simulink model "power_machines_KLFN"  (R2014a)
settings: Solver=ode23tb  SolverMode=SingleTasking  StartTime=0.0  StopTime=60  RelTol=1e-4
libraries: powerlib x17, simulink x3, spsAC1AModel x3, powerlib_meascontrol x1
Description:
  | Copyright 2008-2014 The MathWorks, Inc.
settings Model: FPTRunName=Active  ExtModeTrigMode=oneshot  ExtModeArmWhenConnect=off  ExtModeAutoUpdateStatusClock=off  Creator=MathWorks  LastModifiedBy=jdlara
settings SolverCC: ZeroCrossAlgorithm=Adaptive
settings DataIOCC: LimitDataPoints=off  SignalLoggingSaveFormat=ModelDataLogs  SignalLoggingName=sigsOut  OutputTimes=[0:1/20:10]
settings OptimizationCC: BlockReduction=off  BooleanDataType=off  ExpressionDepthLimit=2147483647  InitFltsAndDblsToZero=on  EfficientMapNaN2IntZero=off
settings DebuggingCC: UnderspecifiedInitializationDetection=Classic  CheckExecutionContextPreStartOutputMsg=on  CheckExecutionContextRuntimeOutputMsg=on  SignalResolutionControl=TryResolveAllWithWarning  IgnoredZcDiagnostic=none  SolverPrmCheckMsg=none  MultiTaskDSMMsg=warning  MultiTaskCondExecSysMsg=none  SigSpecEnsureSampleTimeMsg=none  FcnCallInpInsideContextMsg=UseLocalSettings  UnconnectedInputMsg=none  UnconnectedOutputMsg=none  UnconnectedLineMsg=none  StateNameClashWarn=warning
settings HardwareCC: ProdHWDeviceType=Specified  TargetUnknown=on
settings RTWCC: IncludeERTFirstTime=on
settings CodeAppCC: IgnoreCustomStorageClasses=off
settings GRTTargetCC: TargetFcnLib=ansi_tfl_tmw.mat  CombineOutputUpdateFcns=off  GRTInterface=on

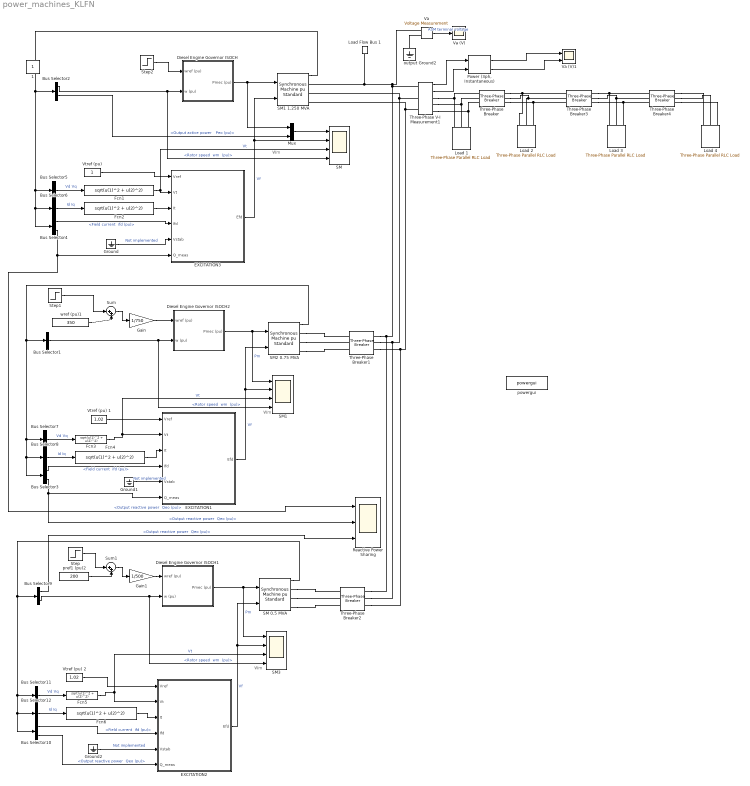
== system power_machines_KLFN ==
  note: Wm
  note: Wm
  note: Wm
  Bus Selector1 : BusSelector  OutputSignals="Mechanical.Rotor speed  wm  (pu)"
  Bus Selector10 : BusSelector  OutputSignals="dq0 components.Field current  ifd (pu),Output reactive power  Qeo (pu)"
  Bus Selector11 : BusSelector  OutputSignals="dq0 components.Stator voltage  vd (pu),dq0 components.Stator voltage  vq (pu)"  OutputAsBus=on
  Bus Selector12 : BusSelector  OutputSignals="dq0 components.Stator current  id (pu),dq0 components.Stator current  iq (pu)"  OutputAsBus=on
  Bus Selector2 : BusSelector  OutputSignals="Mechanical.Rotor speed  wm  (pu),Output active power   Peo (pu)"
  Bus Selector3 : BusSelector  OutputSignals="dq0 components.Field current  ifd (pu),Output reactive power  Qeo (pu)"
  Bus Selector4 : BusSelector  OutputSignals="dq0 components.Field current  ifd (pu),Output reactive power  Qeo (pu)"
  Bus Selector5 : BusSelector  OutputSignals="dq0 components.Stator voltage  vd (pu),dq0 components.Stator voltage  vq (pu)"  OutputAsBus=on
  Bus Selector6 : BusSelector  OutputSignals="dq0 components.Stator current  id (pu),dq0 components.Stator current  iq (pu)"  OutputAsBus=on
  Bus Selector7 : BusSelector  OutputSignals="dq0 components.Stator voltage  vd (pu),dq0 components.Stator voltage  vq (pu)"  OutputAsBus=on
  Bus Selector8 : BusSelector  OutputSignals="dq0 components.Stator current  id (pu),dq0 components.Stator current  iq (pu)"  OutputAsBus=on
  Bus Selector9 : BusSelector  OutputSignals="Output reactive power  Qeo (pu),Mechanical.Rotor speed  wm  (pu)"
  Diesel Engine Governor ISOCH : Subsystem  mask(Diesel Engine & Governor){K=5, Tr=[0.018 0.001 0.38], Ta=[0.35 0.002 0.015], Tlim=[0 1.2], Td=0.024, Pm0=0.58197}
      mask prompts: K "Regulator gain K:"; Tr "Regulator time constants [T1 T2 T3 ] (s) :"; Ta "Actuator time constants [T4 T5 T6] (s) :"; Tlim "Torque limits [Tmin Tmax] (pu) :"; Td "Engine time delay Td (s) :"; Pm0 "Initial value of mechanical power  Pm0 (pu) :"
      mask help:
      | This block implements a diesel engine and governor system:
      | 1st and 2nd inputs: Desired and actual speed (pu)
      | Output: Diesel engine mechanical power.Motor inertia should be combined with generator.
      | Controller transfer function:
      |      Hc=K.(1+T3.s)/(1+T1.s+T1.T2.s^2)
      | Actuator transfer function :
      |      Ha= (1+T4.s) / [ (s (1+T5.s)(1+T6.s) ]
      | Motor :
      |      Time delay Td
      |
      | (See reference in Tutorial Session 5)
  Diesel Engine Governor ISOCH1 : Subsystem  mask(Diesel Engine & Governor){K=5, Tr=[0.018 0.001 0.38], Ta=[0.35 0.002 0.015], Tlim=[0 1.2], Td=0.024, Pm0=0.40148}
      mask prompts: K "Regulator gain K:"; Tr "Regulator time constants [T1 T2 T3 ] (s) :"; Ta "Actuator time constants [T4 T5 T6] (s) :"; Tlim "Torque limits [Tmin Tmax] (pu) :"; Td "Engine time delay Td (s) :"; Pm0 "Initial value of mechanical power  Pm0 (pu) :"
      mask help:
      | This block implements a diesel engine and governor system:
      | 1st and 2nd inputs: Desired and actual speed (pu)
      | Output: Diesel engine mechanical power.Motor inertia should be combined with generator.
      | Controller transfer function:
      |      Hc=K.(1+T3.s)/(1+T1.s+T1.T2.s^2)
      | Actuator transfer function :
      |      Ha= (1+T4.s) / [ (s (1+T5.s)(1+T6.s) ]
      | Motor :
      |      Time delay Td
      |
      | (See reference in Tutorial Session 5)
  Diesel Engine Governor ISOCH2 : Subsystem  mask(Diesel Engine & Governor){K=5, Tr=[0.018 0.001 0.38], Ta=[0.35 0.002 0.015], Tlim=[0 1.2], Td=0.024, Pm0=0.46784}
      mask prompts: K "Regulator gain K:"; Tr "Regulator time constants [T1 T2 T3 ] (s) :"; Ta "Actuator time constants [T4 T5 T6] (s) :"; Tlim "Torque limits [Tmin Tmax] (pu) :"; Td "Engine time delay Td (s) :"; Pm0 "Initial value of mechanical power  Pm0 (pu) :"
      mask help:
      | This block implements a diesel engine and governor system:
      | 1st and 2nd inputs: Desired and actual speed (pu)
      | Output: Diesel engine mechanical power.Motor inertia should be combined with generator.
      | Controller transfer function:
      |      Hc=K.(1+T3.s)/(1+T1.s+T1.T2.s^2)
      | Actuator transfer function :
      |      Ha= (1+T4.s) / [ (s (1+T5.s)(1+T6.s) ]
      | Motor :
      |      Time delay Td
      |
      | (See reference in Tutorial Session 5)
  EXCITATION1 : Subsystem  Variant=on  OverrideUsingVariant=Variant1
      settings: AttributesFormatString=%<BlockChoice>
  EXCITATION2 : Subsystem  Variant=on  OverrideUsingVariant=Variant1
      settings: AttributesFormatString=%<BlockChoice>
  EXCITATION3 : Subsystem  Variant=on  OverrideUsingVariant=Variant1
      settings: AttributesFormatString=%<BlockChoice>
  Fcn{1..6} (6 alike) : Fcn  Expr=sqrt(u(1)^2 + u(2)^2)
  Gain : Gain  Gain=1/750
  Gain1 : Gain  Gain=1/500
  Ground : Ground
  Ground1 : Ground
  Ground2 : Ground
  Load 1 : powerlib/Elements/Three-Phase Parallel RLC Load  LConnTagsString=A|B|C  Configuration=Y (grounded)  NominalVoltage=600  NominalFrequency=60  ActivePower=10e+005  InductivePower=1.8e5  CapacitivePower=0  Measurements=None  LoadType=constant Z
  Load 2 : powerlib/Elements/Three-Phase Parallel RLC Load  LConnTagsString=A|B|C  Configuration=Y (grounded)  NominalVoltage=600  NominalFrequency=60  ActivePower=2.5e+05  InductivePower=8.8e5  CapacitivePower=0  Measurements=None  LoadType=constant Z
  Load 3 : powerlib/Elements/Three-Phase Parallel RLC Load  LConnTagsString=A|B|C  Configuration=Y (grounded)  NominalVoltage=600  NominalFrequency=60  ActivePower=1.5e+05  InductivePower=2.8e5  CapacitivePower=0  Measurements=None  LoadType=constant Z
  Load 4 : powerlib/Elements/Three-Phase Parallel RLC Load  LConnTagsString=A|B|C  Configuration=Y (grounded)  NominalVoltage=600  NominalFrequency=60  ActivePower=1.5e+05  InductivePower=2.8e5  CapacitivePower=0  Measurements=None  LoadType=constant Z
  Load Flow Bus 1 : powerlib/Measurements/Load Flow Bus  LConnTagsString=a  ID=B2  Vbase=600  Vref=1.0  Vangle=0  VLF=1  angleLF=0
      settings: AttributesFormatString=%<ID>\n%<Vbase>V\n%<VLF>pu\n%<angleLF>deg.
  Mux : Mux  Inputs=2
  "Power (3ph, Instantaneous)" : powerlib_meascontrol/Measurements/Power (3ph, Instantaneous)
  Reactive Power Sharing : Scope  NumInputPorts=3
      settings: TimeRange=60  YMin=-0.175~0.3525~0.4375  YMax=0.075~0.3775~0.46  SaveName=Pmec_SM2  DataFormat=Structure  Decimation=10
  SM : Scope  NumInputPorts=4
      settings: TimeRange=10  YMin=0.801025~2.065~1.0075~0.984429  YMax=0.80145~2.13~1.013~0.984434  SaveName=Pmec_SM1  DataFormat=Structure  Decimation=10
  SM 0.5 MVA : powerlib/Machines/Synchronous Machine pu Standard  PresetModel=No  MechanicalLoad=Mechanical power Pm  ShowDetailedParameters=on  RotorType=Salient-pole  Units=per unit standard parameters  MeasurementBus=off  NominalParameters="[ 0.5e6  600  60]"  Reactances1=[ 31 32 33 34 35 36 37 ]  Reactances2=[ 1.7479, 0.082064, 0.070619, 1.1516, 0.1307, 0.04 ]  dAxisTimeConstants=Short-circuit  qAxisTimeConstants=Short-circuit  TimeConstants1=[]  TimeConstants2=[]  TimeConstants3=[]  TimeConstants4=[]  TimeConstants5=[ 3.7, 0.05, 0.05 ]  TimeConstants6=[ 8.0, 0.03, 0.3371, 0.0295 ]  TimeConstants7=[0.1325 0.0185 0.006]  TimeConstants8=[]  StatorResistance=0.0036  Mechanical="[0.2548  0.01 2]"  PolePairs=2  InitialConditions=[0 -74.3609 0.641948 0.641948 0.641948 -52.1071 -172.107 67.8929 2.00572]  SetSaturation=off  Saturation=[0.211 0.418 1.0 1.25 1.72 3.35 ;0.25 0.50 1.0 1.1 1.2 1.4]  LoadFlowParameters=[4 0 0 0]  TsPowergui=0  TsBlock=-1  IterativeModel=Forward Euler  BusType=PQ  Pref=200e3  Qref=2.533e5  Qmin=-Inf  Qmax=Inf  PLF=0  QLF=0
      settings: AttributesFormatString=\n\n
  SM1 : Scope  NumInputPorts=4
      settings: TimeRange=4.8  YMin=0~0.2~0.5~1.14087  YMax=1.1~0.375~1.1~1.14107  SaveName=Pmec_SM  DataFormat=Structure  Decimation=10
  SM1 1.250 MVA : powerlib/Machines/Synchronous Machine pu Standard  PresetModel=No  MechanicalLoad=Mechanical power Pm  ShowDetailedParameters=on  RotorType=Salient-pole  Units=per unit standard parameters  MeasurementBus=off  NominalParameters="[ 1.25e6  600  60]"  Reactances1=[ 31 32 33 34 35 36 37 ]  Reactances2=[ 1.97, 0.1318, 0.092, 0.96, 0.122, 0.049 ]  dAxisTimeConstants=Short-circuit  qAxisTimeConstants=Short-circuit  TimeConstants1=[]  TimeConstants2=[]  TimeConstants3=[]  TimeConstants4=[]  TimeConstants5=[ 0.185, 0.025, 0.005 ]  TimeConstants6=[ 8.0, 0.03, 0.3371, 0.0295 ]  TimeConstants7=[0.185 0.025 0.006]  TimeConstants8=[]  StatorResistance=0.00036  Mechanical="[0.3134  0.01 2]"  PolePairs=2  InitialConditions=[0 -68.4764 0.725136 0.725136 0.725136 -36.6497 -156.65 83.3503 2.14414]  SetSaturation=off  Saturation=[0.211 0.418 1.0 1.25 1.72 3.35 ;0.25 0.50 1.0 1.1 1.2 1.4]  LoadFlowParameters=[2 0 0 0]  TsPowergui=0  TsBlock=-1  IterativeModel=Forward Euler  BusType=swing  Pref=0  Qref=0  Qmin=-Inf  Qmax=Inf  PLF=0  QLF=0
      settings: AttributesFormatString=\n\n
  SM2 0.75 MVA : powerlib/Machines/Synchronous Machine pu Standard  PresetModel=No  MechanicalLoad=Mechanical power Pm  ShowDetailedParameters=on  RotorType=Salient-pole  Units=per unit standard parameters  MeasurementBus=off  NominalParameters="[0.75e6  600  60]"  Reactances1=[ 31 32 33 34 35 36 37 ]  Reactances2=[ 1.748873, 0.07546, 0.052043, 1.256839, 0.1483, 0.026]  dAxisTimeConstants=Short-circuit  qAxisTimeConstants=Short-circuit  TimeConstants1=[]  TimeConstants2=[]  TimeConstants3=[]  TimeConstants4=[]  TimeConstants5=[ 3.7, 0.05, 0.05 ]  TimeConstants6=[ 8.0, 0.03, 0.3371, 0.0295 ]  TimeConstants7=[0.08 0.012 0.006]  TimeConstants8=[]  StatorResistance=0.0036  Mechanical="[0.2186  0.001 2]"  PolePairs=2  InitialConditions=[0 -68.3474 0.570344 0.570344 0.570344 -36.2604 -156.26 83.7396 1.78193]  SetSaturation=off  Saturation=[0.211 0.418 1.0 1.25 1.72 3.35 ;0.25 0.50 1.0 1.1 1.2 1.4]  LoadFlowParameters=[4 0 0 0]  TsPowergui=0  TsBlock=-1  IterativeModel=Forward Euler  BusType=PQ  Pref=350e3  Qref=2.53e5  Qmin=-Inf  Qmax=Inf  PLF=0  QLF=0
      settings: AttributesFormatString=\n\n
  SM3 : Scope  NumInputPorts=4
      settings: TimeRange=4.8  YMin=0.3~0.3975~1.04425~0.994  YMax=1.1~0.4175~1.04575~0.998  SaveName=Pmec_SM3  DataFormat=Structure  Decimation=10
  Step : Step  Time=30.5  After=120  SampleTime=0
  Step1 : Step  Time=20.5  After=150  SampleTime=0
  Step2 : Step  Before=1.0  After=1.1  SampleTime=0
  Sum : Sum  Inputs=|++
  Sum1 : Sum  Inputs=|++
  Three-Phase V-I Measurement1 : powerlib/Measurements/Three-Phase V-I Measurement  VoltageMeasurement=phase-to-phase  SetLabelV=off  LabelV=Vabc  Vpu=off  VpuLL=off  CurrentMeasurement=yes  SetLabelI=off  LabelI=Iabc  Ipu=off  Pbase=100e6  Vbase=(2400)*1/sqrt(2)  OutputType=Complex  PhasorSimulation=off  PSBequivalent=0
  Three-Phase Breaker : powerlib/Elements/Three-Phase Breaker  InitialState=closed  SwitchA=on  SwitchB=on  SwitchC=on  SwitchTimes=100  External=off  BreakerResistance=0.01  SnubberResistance=1e6  SnubberCapacitance=inf  Measurements=None
  Three-Phase Breaker1 : powerlib/Elements/Three-Phase Breaker  InitialState=closed  SwitchA=on  SwitchB=on  SwitchC=on  SwitchTimes=[149.9]  External=off  BreakerResistance=0.01  SnubberResistance=1e6  SnubberCapacitance=inf  Measurements=None
  Three-Phase Breaker2 : powerlib/Elements/Three-Phase Breaker  InitialState=closed  SwitchA=on  SwitchB=on  SwitchC=on  SwitchTimes="[150  270]"  External=off  BreakerResistance=0.01  SnubberResistance=1e6  SnubberCapacitance=inf  Measurements=None
  Three-Phase Breaker3 : powerlib/Elements/Three-Phase Breaker  InitialState=open  SwitchA=on  SwitchB=on  SwitchC=on  SwitchTimes=[20]  External=off  BreakerResistance=0.01  SnubberResistance=1e6  SnubberCapacitance=inf  Measurements=None
  Three-Phase Breaker4 : powerlib/Elements/Three-Phase Breaker  InitialState=open  SwitchA=on  SwitchB=on  SwitchC=on  SwitchTimes=[30]  External=off  BreakerResistance=0.01  SnubberResistance=1e6  SnubberCapacitance=inf  Measurements=None
  Va : powerlib/Measurements/Voltage Measurement  Tag=PoWeRsYsTeMmEaSuReMeNt  PhasorSimulation=off  OutputType=Magnitude  PSBequivalent=0
  Va (V) : Scope
      settings: TickLabels=on  TimeRange=5  YMin=-500  YMax=500
  Va (V)1 : Scope  NumInputPorts=2
      settings: TickLabels=on  TimeRange=5  YMin=0.0086265~-5  YMax=0.00862875~5  SaveName=ScopeData2
  "Vtref (pu) " : Constant
  Vtref (pu) 1 : Constant  Value=1.02
  Vtref (pu) 2 : Constant  Value=1.02
  output Ground2 : powerlib/Elements/Ground  LConnTagsString=a
  powergui : powerlib/powergui  Priority=2  SimulationMode=Continuous  SolverType=Tustin  SampleTime=50e-6  frequency=60  SPID=off  DisableSnubberDevices=off  DisableRonSwitches=off  DisableVfSwitches=off  SwTol=0  Interpol=off  DisplayEquations=off  Ts=0  methode=off  frequencyindice=60  Pbase=1e6  ErrMax=0.0001  Iterations=50  UnitsV=kV  UnitsW=MW  FunctionMessages=off  echomessages=off  HookPort=off  EnableUseOfTLC=off  x0status=blocks  RestoreLinks=warning  ResistiveCurrentMeasurement=off  Frange=logspace(0,3,50)  Ylog=off  Xlog=off  ShowGrid=off  save=off  variable=ZData  structure=0  ZoomFFT=on  StartTime=0.0  cycles=2  DisplayStyle=off  fundamental=60  FreqAxis=off  MaxFrequency=1000  frequencyindicesteady=1  RmsSteady=1  display=off
  pref1 (pu)2 : Constant  Value=200
  wref (pu)1 : Constant  Value=350
  1 : Constant  IOType=siggen
  wires:
  Va/1 -> Va (V)/1  "ASM terminal voltage"
  Diesel Engine Governor ISOCH/1(Pmec (pu)) -> Mux/1, SM1 1.250 MVA/1
  Fcn2/1 -> EXCITATION3/3(It)
  Bus Selector4/1 -> EXCITATION3/4(Ifd)  "<Field current  ifd (pu)>"
  Bus Selector6/1 -> Fcn2/1  "Id Iq"
  Ground/1 -> EXCITATION3/5(Vstab)  "Not implemented"
  Bus Selector5/1 -> Fcn1/1  "Vd Vq"
  Bus Selector2/1 -> Diesel Engine Governor ISOCH/2(w (pu)), SM/4  "<Rotor speed  wm  (pu)>"
  Fcn1/1 -> SM/3, EXCITATION3/2(Vt)  "Vt"
  EXCITATION3/1(Efd) -> SM1 1.250 MVA/2, SM/2  "Vf"
  "Vtref (pu) "/1 -> EXCITATION3/1(Vref)
  SM1 1.250 MVA/1 -> Bus Selector2/1, Bus Selector5/1, Bus Selector6/1, Bus Selector4/1
  Diesel Engine Governor ISOCH2/1(Pmec (pu)) -> SM1/1, SM2 0.75 MVA/1  "Pm"
  Fcn4/1 -> EXCITATION1/3(It)
  Bus Selector3/1 -> EXCITATION1/4(Ifd)  "<Field current  ifd (pu)>"
  Bus Selector8/1 -> Fcn4/1  "Id Iq"
  Ground1/1 -> EXCITATION1/5(Vstab)  "Not implemented"
  Bus Selector7/1 -> Fcn3/1  "Vd Vq"
  Bus Selector1/1 -> Diesel Engine Governor ISOCH2/2(w (pu)), SM1/4  "<Rotor speed  wm  (pu)>"
  Fcn3/1 -> EXCITATION1/2(Vt), SM1/3  "Vt"
  EXCITATION1/1(Efd) -> SM1/2, SM2 0.75 MVA/2  "Vf"
  Vtref (pu) 1/1 -> EXCITATION1/1(Vref)
  SM2 0.75 MVA/1 -> Bus Selector1/1, Bus Selector7/1, Bus Selector8/1, Bus Selector3/1
  Bus Selector4/2 -> EXCITATION3/6(Q_meas), Reactive Power Sharing/1  "<Output reactive power  Qeo (pu)>"
  Diesel Engine Governor ISOCH1/1(Pmec (pu)) -> SM3/1, SM 0.5 MVA/1  "Pm"
  Fcn6/1 -> EXCITATION2/3(It)
  Bus Selector10/1 -> EXCITATION2/4(Ifd)  "<Field current  ifd (pu)>"
  Bus Selector12/1 -> Fcn6/1  "Id Iq"
  Ground2/1 -> EXCITATION2/5(Vstab)  "Not implemented"
  Bus Selector11/1 -> Fcn5/1  "Vd Vq"
  Bus Selector9/2 -> Diesel Engine Governor ISOCH1/2(w (pu)), SM3/4  "<Rotor speed  wm  (pu)>"
  Fcn5/1 -> EXCITATION2/2(Vt), SM3/3  "Vt"
  EXCITATION2/1(Efd) -> SM3/2, SM 0.5 MVA/2  "Vf"
  Vtref (pu) 2/1 -> EXCITATION2/1(Vref)
  SM 0.5 MVA/1 -> Bus Selector9/1, Bus Selector11/1, Bus Selector12/1, Bus Selector10/1
  Bus Selector9/1 -> Reactive Power Sharing/3  "<Output reactive power  Qeo (pu)>"
  Bus Selector3/2 -> EXCITATION1/6(Q_meas), Reactive Power Sharing/2  "<Output reactive power  Qeo (pu)>"
  Bus Selector10/2 -> EXCITATION2/6(Q_meas)  "<Output reactive power  Qeo (pu)>"
  Gain/1 -> Diesel Engine Governor ISOCH2/1(wref (pu))
  Gain1/1 -> Diesel Engine Governor ISOCH1/1(wref (pu))
  wref (pu)1/1 -> Sum/2
  Sum/1 -> Gain/1
  pref1 (pu)2/1 -> Sum1/2
  Sum1/1 -> Gain1/1
  Step/1 -> Sum1/1
  Step1/1 -> Sum/1
  Three-Phase V-I Measurement1/1 -> "Power (3ph, Instantaneous)"/1
  Three-Phase V-I Measurement1/2 -> "Power (3ph, Instantaneous)"/2
  "Power (3ph, Instantaneous)"/1 -> Va (V)1/1
  "Power (3ph, Instantaneous)"/2 -> Va (V)1/2
  Step2/1 -> Diesel Engine Governor ISOCH/1(wref (pu))
  Mux/1 -> SM/1
  Bus Selector2/2 -> Mux/2  "<Output active power   Peo (pu)>"
  connections:
  output Ground2/LConn1 -- Va/LConn2
  Three-Phase Breaker/LConn2 -- Three-Phase V-I Measurement1/RConn2 -- Load 1/LConn2
  Three-Phase Breaker/LConn1 -- Three-Phase V-I Measurement1/RConn1 -- Load 1/LConn1
  Load 1/LConn3 -- Three-Phase V-I Measurement1/RConn3 -- Three-Phase Breaker/LConn3
  Three-Phase Breaker/RConn1 -- Three-Phase Breaker3/LConn1 -- Load 2/LConn1
  Three-Phase Breaker/RConn2 -- Three-Phase Breaker3/LConn2 -- Load 2/LConn2
  Three-Phase Breaker/RConn3 -- Three-Phase Breaker3/LConn3 -- Load 2/LConn3
  SM2 0.75 MVA/RConn1 -- Three-Phase Breaker1/LConn1
  SM2 0.75 MVA/RConn2 -- Three-Phase Breaker1/LConn2
  SM2 0.75 MVA/RConn3 -- Three-Phase Breaker1/LConn3
  SM 0.5 MVA/RConn1 -- Three-Phase Breaker2/LConn1
  SM 0.5 MVA/RConn3 -- Three-Phase Breaker2/LConn3
  SM 0.5 MVA/RConn2 -- Three-Phase Breaker2/LConn2
  Three-Phase Breaker3/RConn2 -- Three-Phase Breaker4/LConn2 -- Load 3/LConn2
  Three-Phase Breaker3/RConn1 -- Three-Phase Breaker4/LConn1 -- Load 3/LConn1
  Three-Phase Breaker3/RConn3 -- Three-Phase Breaker4/LConn3 -- Load 3/LConn3
  Three-Phase Breaker4/RConn2 -- Load 4/LConn2
  Three-Phase Breaker4/RConn1 -- Load 4/LConn1
  Three-Phase Breaker4/RConn3 -- Load 4/LConn3
  Three-Phase Breaker1/RConn2 -- Three-Phase V-I Measurement1/LConn2 -- SM1 1.250 MVA/RConn2 -- Three-Phase Breaker2/RConn2
  Three-Phase Breaker2/RConn1 -- Va/LConn1 -- SM1 1.250 MVA/RConn1 -- Load Flow Bus 1/LConn1 -- Three-Phase V-I Measurement1/LConn1 -- Three-Phase Breaker1/RConn1
  Three-Phase Breaker2/RConn3 -- Three-Phase V-I Measurement1/LConn3 -- SM1 1.250 MVA/RConn3 -- Three-Phase Breaker1/RConn3

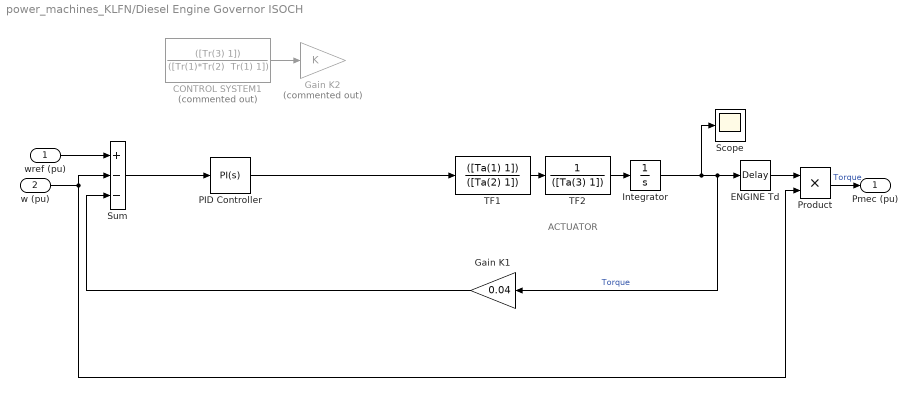
== system power_machines_KLFN/Diesel Engine Governor ISOCH ==
  note: ACTUATOR
  wref (pu) : Inport
  w (pu) : Inport  Port=2
  CONTROL SYSTEM1 : TransferFcn  Commented=on  Numerator=([Tr(3) 1])  Denominator="([Tr(1)*Tr(2)  Tr(1) 1])"
  ENGINE Td : TransportDelay  DelayTime=Td  InitialOutput=Pm0
  Gain K1 : Gain  Gain=0.04  SaturateOnIntegerOverflow=on  OutDataTypeStr=Inherit: Same as input  ParamDataTypeStr=Inherit: Same as input
  Gain K2 : Gain  Commented=on  Gain=K  SaturateOnIntegerOverflow=on  OutDataTypeStr=Inherit: Same as input  ParamDataTypeStr=Inherit: Same as input
  Integrator : Integrator  InitialCondition=Pm0  LimitOutput=on  UpperSaturationLimit=Tlim(2)  LowerSaturationLimit=Tlim(1)
  PID Controller : simulink/Continuous/PID Controller  Controller=PI  TimeDomain=Continuous-time  SampleTime=1  IntegratorMethod=Forward Euler  FilterMethod=Forward Euler  Form=Parallel  P=30  I=75  D=0  N=0  InitialConditionSource=internal  InitialConditionForIntegrator=0  InitialConditionForFilter=0  ExternalReset=none  LimitOutput=off  UpperSaturationLimit=inf  LowerSaturationLimit=-inf  LinearizeAsGain=on  AntiWindupMode=none  Kb=1  TrackingMode=off  Kt=1  PParamMin=[]  PParamMax=[]  IParamMin=[]  IParamMax=[]  DParamMin=[]  DParamMax=[]  NParamMin=[]  NParamMax=[]  KbParamMin=[]  KbParamMax=[]  KtParamMin=[]  KtParamMax=[]  POutMin=[]  POutMax=[]  IOutMin=[]  IOutMax=[]  DOutMin=[]  DOutMax=[]  NOutMin=[]  NOutMax=[]  KbOutMin=[]  KbOutMax=[]  KtOutMin=[]  KtOutMax=[]  IntegratorOutMin=[]  IntegratorOutMax=[]  FilterOutMin=[]  FilterOutMax=[]  SumOutMin=[]  SumOutMax=[]  SumI1OutMin=[]  SumI1OutMax=[]  SumI2OutMin=[]  SumI2OutMax=[]  SumI3OutMin=[]  SumI3OutMax=[]  SumDOutMin=[]  SumDOutMax=[]  SaturationOutMin=[]  SaturationOutMax=[]  IntegratorContinuousStateAttributes=''  IntegratorStateMustResolveToSignalObject=off  IntegratorRTWStateStorageClass=Auto  FilterContinuousStateAttributes=''  FilterStateMustResolveToSignalObject=off  FilterRTWStateStorageClass=Auto
  Product : Product  SaturateOnIntegerOverflow=on  InputSameDT=on  OutDataTypeStr=Inherit: Same as first input
  Scope : Scope
      settings: Decimation=10
  Sum : Sum  Inputs=+--  SaturateOnIntegerOverflow=on  InputSameDT=on  OutDataTypeStr=Inherit: Same as first input
  TF1 : TransferFcn  Numerator=([Ta(1) 1])  Denominator=([Ta(2) 1])
  TF2 : TransferFcn  Numerator=1  Denominator=([Ta(3) 1])
  Pmec (pu) : Outport  InitialOutput=0
  wires:
  Integrator/1 -> Scope/1, Gain K1/1, ENGINE Td/1  "Torque"
  TF2/1 -> Integrator/1
  wref (pu)/1 -> Sum/1
  ENGINE Td/1 -> Product/1
  w (pu)/1 -> Sum/2, Product/2
  TF1/1 -> TF2/1
  Sum/1 -> PID Controller/1
  PID Controller/1 -> TF1/1
  Gain K1/1 -> Sum/3
  Product/1 -> Pmec (pu)/1  "Torque"
  CONTROL SYSTEM1/1 -> Gain K2/1

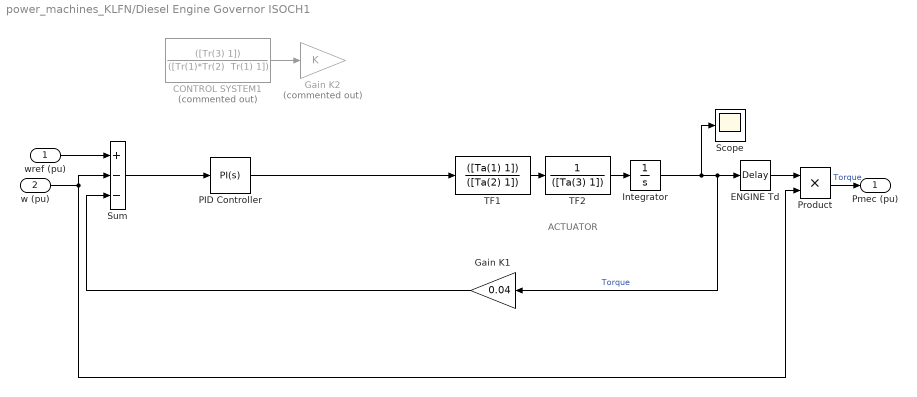
== system power_machines_KLFN/Diesel Engine Governor ISOCH1 ==
  note: ACTUATOR
  wref (pu) : Inport
  w (pu) : Inport  Port=2
  CONTROL SYSTEM1 : TransferFcn  Commented=on  Numerator=([Tr(3) 1])  Denominator="([Tr(1)*Tr(2)  Tr(1) 1])"
  ENGINE Td : TransportDelay  DelayTime=Td  InitialOutput=Pm0
  Gain K1 : Gain  Gain=0.04  SaturateOnIntegerOverflow=on  OutDataTypeStr=Inherit: Same as input  ParamDataTypeStr=Inherit: Same as input
  Gain K2 : Gain  Commented=on  Gain=K  SaturateOnIntegerOverflow=on  OutDataTypeStr=Inherit: Same as input  ParamDataTypeStr=Inherit: Same as input
  Integrator : Integrator  InitialCondition=Pm0  LimitOutput=on  UpperSaturationLimit=Tlim(2)  LowerSaturationLimit=Tlim(1)
  PID Controller : simulink/Continuous/PID Controller  Controller=PI  TimeDomain=Continuous-time  SampleTime=1  IntegratorMethod=Forward Euler  FilterMethod=Forward Euler  Form=Parallel  P=30  I=75  D=0  N=0  InitialConditionSource=internal  InitialConditionForIntegrator=0  InitialConditionForFilter=0  ExternalReset=none  LimitOutput=off  UpperSaturationLimit=inf  LowerSaturationLimit=-inf  LinearizeAsGain=on  AntiWindupMode=none  Kb=1  TrackingMode=off  Kt=1  PParamMin=[]  PParamMax=[]  IParamMin=[]  IParamMax=[]  DParamMin=[]  DParamMax=[]  NParamMin=[]  NParamMax=[]  KbParamMin=[]  KbParamMax=[]  KtParamMin=[]  KtParamMax=[]  POutMin=[]  POutMax=[]  IOutMin=[]  IOutMax=[]  DOutMin=[]  DOutMax=[]  NOutMin=[]  NOutMax=[]  KbOutMin=[]  KbOutMax=[]  KtOutMin=[]  KtOutMax=[]  IntegratorOutMin=[]  IntegratorOutMax=[]  FilterOutMin=[]  FilterOutMax=[]  SumOutMin=[]  SumOutMax=[]  SumI1OutMin=[]  SumI1OutMax=[]  SumI2OutMin=[]  SumI2OutMax=[]  SumI3OutMin=[]  SumI3OutMax=[]  SumDOutMin=[]  SumDOutMax=[]  SaturationOutMin=[]  SaturationOutMax=[]  IntegratorContinuousStateAttributes=''  IntegratorStateMustResolveToSignalObject=off  IntegratorRTWStateStorageClass=Auto  FilterContinuousStateAttributes=''  FilterStateMustResolveToSignalObject=off  FilterRTWStateStorageClass=Auto
  Product : Product  SaturateOnIntegerOverflow=on  InputSameDT=on  OutDataTypeStr=Inherit: Same as first input
  Scope : Scope
      settings: Decimation=10
  Sum : Sum  Inputs=+--  SaturateOnIntegerOverflow=on  InputSameDT=on  OutDataTypeStr=Inherit: Same as first input
  TF1 : TransferFcn  Numerator=([Ta(1) 1])  Denominator=([Ta(2) 1])
  TF2 : TransferFcn  Numerator=1  Denominator=([Ta(3) 1])
  Pmec (pu) : Outport  InitialOutput=0
  wires:
  Integrator/1 -> Scope/1, Gain K1/1, ENGINE Td/1  "Torque"
  TF2/1 -> Integrator/1
  wref (pu)/1 -> Sum/1
  ENGINE Td/1 -> Product/1
  w (pu)/1 -> Sum/2, Product/2
  TF1/1 -> TF2/1
  Sum/1 -> PID Controller/1
  PID Controller/1 -> TF1/1
  Gain K1/1 -> Sum/3
  Product/1 -> Pmec (pu)/1  "Torque"
  CONTROL SYSTEM1/1 -> Gain K2/1

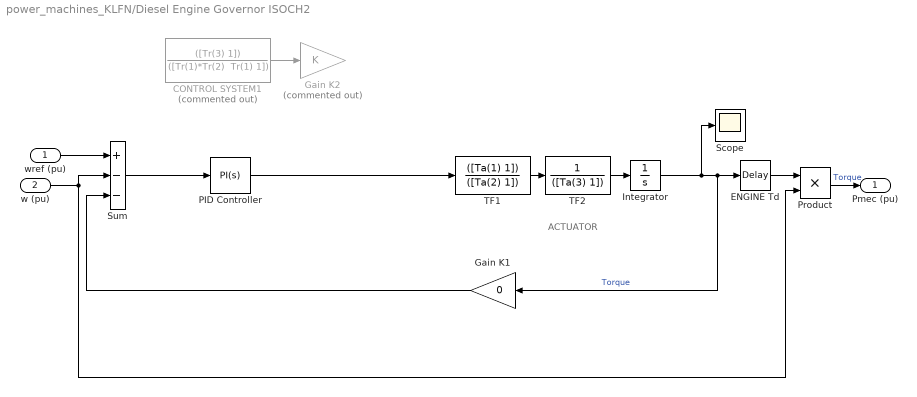
== system power_machines_KLFN/Diesel Engine Governor ISOCH2 ==
  note: ACTUATOR
  wref (pu) : Inport
  w (pu) : Inport  Port=2
  CONTROL SYSTEM1 : TransferFcn  Commented=on  Numerator=([Tr(3) 1])  Denominator="([Tr(1)*Tr(2)  Tr(1) 1])"
  ENGINE Td : TransportDelay  DelayTime=Td  InitialOutput=Pm0
  Gain K1 : Gain  Gain=0  SaturateOnIntegerOverflow=on  OutDataTypeStr=Inherit: Same as input  ParamDataTypeStr=Inherit: Same as input
  Gain K2 : Gain  Commented=on  Gain=K  SaturateOnIntegerOverflow=on  OutDataTypeStr=Inherit: Same as input  ParamDataTypeStr=Inherit: Same as input
  Integrator : Integrator  InitialCondition=Pm0  LimitOutput=on  UpperSaturationLimit=Tlim(2)  LowerSaturationLimit=Tlim(1)
  PID Controller : simulink/Continuous/PID Controller  Controller=PI  TimeDomain=Continuous-time  SampleTime=1  IntegratorMethod=Forward Euler  FilterMethod=Forward Euler  Form=Parallel  P=30  I=75  D=0  N=0  InitialConditionSource=internal  InitialConditionForIntegrator=0  InitialConditionForFilter=0  ExternalReset=none  LimitOutput=off  UpperSaturationLimit=inf  LowerSaturationLimit=-inf  LinearizeAsGain=on  AntiWindupMode=none  Kb=1  TrackingMode=off  Kt=1  PParamMin=[]  PParamMax=[]  IParamMin=[]  IParamMax=[]  DParamMin=[]  DParamMax=[]  NParamMin=[]  NParamMax=[]  KbParamMin=[]  KbParamMax=[]  KtParamMin=[]  KtParamMax=[]  POutMin=[]  POutMax=[]  IOutMin=[]  IOutMax=[]  DOutMin=[]  DOutMax=[]  NOutMin=[]  NOutMax=[]  KbOutMin=[]  KbOutMax=[]  KtOutMin=[]  KtOutMax=[]  IntegratorOutMin=[]  IntegratorOutMax=[]  FilterOutMin=[]  FilterOutMax=[]  SumOutMin=[]  SumOutMax=[]  SumI1OutMin=[]  SumI1OutMax=[]  SumI2OutMin=[]  SumI2OutMax=[]  SumI3OutMin=[]  SumI3OutMax=[]  SumDOutMin=[]  SumDOutMax=[]  SaturationOutMin=[]  SaturationOutMax=[]  IntegratorContinuousStateAttributes=''  IntegratorStateMustResolveToSignalObject=off  IntegratorRTWStateStorageClass=Auto  FilterContinuousStateAttributes=''  FilterStateMustResolveToSignalObject=off  FilterRTWStateStorageClass=Auto
  Product : Product  SaturateOnIntegerOverflow=on  InputSameDT=on  OutDataTypeStr=Inherit: Same as first input
  Scope : Scope
      settings: Decimation=10
  Sum : Sum  Inputs=+--  SaturateOnIntegerOverflow=on  InputSameDT=on  OutDataTypeStr=Inherit: Same as first input
  TF1 : TransferFcn  Numerator=([Ta(1) 1])  Denominator=([Ta(2) 1])
  TF2 : TransferFcn  Numerator=1  Denominator=([Ta(3) 1])
  Pmec (pu) : Outport  InitialOutput=0
  wires:
  Integrator/1 -> Scope/1, Gain K1/1, ENGINE Td/1  "Torque"
  TF2/1 -> Integrator/1
  wref (pu)/1 -> Sum/1
  ENGINE Td/1 -> Product/1
  w (pu)/1 -> Sum/2, Product/2
  TF1/1 -> TF2/1
  Sum/1 -> PID Controller/1
  PID Controller/1 -> TF1/1
  Gain K1/1 -> Sum/3
  Product/1 -> Pmec (pu)/1  "Torque"
  CONTROL SYSTEM1/1 -> Gain K2/1

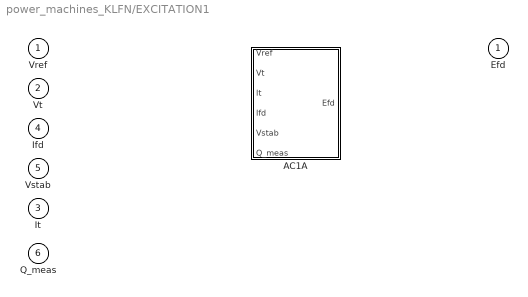
== system power_machines_KLFN/EXCITATION1 ==
  Vref : Inport
  Vt : Inport  Port=2
  It : Inport  Port=3
  Ifd : Inport  Port=4
  Vstab : Inport  Port=5
  Q_meas : Inport  Port=6
  AC1A : Subsystem  VariantControl=Variant1
  Efd : Outport

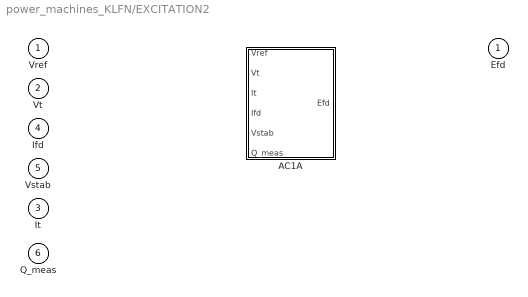
== system power_machines_KLFN/EXCITATION2 ==
  Vref : Inport
  Vt : Inport  Port=2
  It : Inport  Port=3
  Ifd : Inport  Port=4
  Vstab : Inport  Port=5
  Q_meas : Inport  Port=6
  AC1A : Subsystem  VariantControl=Variant1
  Efd : Outport

== system power_machines_KLFN/EXCITATION3 ==
  Vref : Inport
  Vt : Inport  Port=2
  It : Inport  Port=3
  Ifd : Inport  Port=4
  Vstab : Inport  Port=5
  Q_meas : Inport  Port=6
  AC1A : Subsystem  VariantControl=Variant1
  Efd : Outport

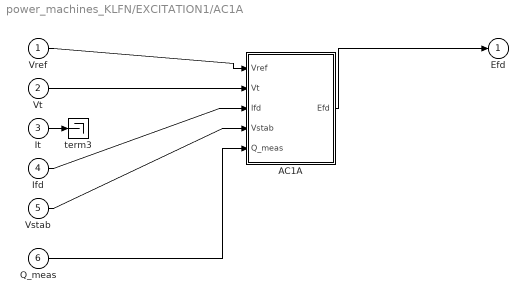
== system power_machines_KLFN/EXCITATION1/AC1A ==
  Vref : Inport
  Vt : Inport  Port=2
  It : Inport  Port=3
  Ifd : Inport  Port=4
  Vstab : Inport  Port=5
  Q_meas : Inport  Port=6
  AC1A : Subsystem  AncestorBlock=sps_avr/AC1A Excitation System  mask(AC1A Excitation System){Tr=20e-11, KaTa=[150 0.012], VAminmax=[-14.5 14.5], VRminmax=[-5.43 6.03], KfTf=[0.03 1.0], TbTc=[0 0], KeTe=[1.0 0.42], Ve12=[4.18 3.14], SeVe12=[0.10 0.03], Kd=0.38, Kc=0.20, v0=[1.0096 1.7819], TsBlock=-2}
      mask prompts: Tr "Low-pass filter time constant Tr(s):"; KaTa "Voltage regulator gain and time constant [Ka Ta(s)]:"; VAminmax "Voltage regulator internal limits [VAmin(pu) VAmax(pu)]:"; VRminmax "Voltage regulator output limits [VRmin(pu) VRmax(pu)]:"; KfTf "Damping filter gain and time constant [Kf Tf(s)]:"; TbTc "Transient gain reduction lead and lag time constants [Tb(s) Tc(s)]:"; KeTe "Exciter gain and time constant [Ke Te(s)]:"; Ve12 "Exciter alternator voltage values [Ve1(pu) Ve2(pu)]:"; SeVe12 "Exciter saturation function values [SeVe1(pu) SeVe2(pu)]:"; Kd "Demagnetizing factor Kd(pu):"; Kc "Rectifier loading factor Kc(pu):"; v0 "Initial values of terminal voltage and field voltage [Vt0(pu) Efd0(pu)]:"; TsBlock "Sample time:"
      mask help: Implements a synchronous machine voltage regulator and exciter based on the IEEE type AC1A excitation system model. The output is the field voltage to apply to the Vf input of a Synchronous Machine block. Inputs and output are in p.u.
      mask init:
      | block = gcb;
      | [Ts,BlockChoice,MaskType,Ka,Ta,Ke,Te,Kf,Tf,Tb,Tc,Ve1,Ve2,SeVe1,SeVe2,VRmin,VRmax,VAmin,VAmax,Ifd0,Ve0,Vfe0,Vt0,Efd0] = powericon('ExcitationSystemInit',block,TsBlock,KaTa,KeTe,KfTf,TbTc,Ve12,SeVe12,VRminmax,VAminmax,Kc,Kd,v0);
      | powericon('SetInternalModels','set',block,BlockChoice);
      mask Help: helpview(psbhelp);
      mask Display: color('blue');disp('AC1A')
  term3 : Terminator
  Efd : Outport
  wires:
  It/1 -> term3/1
  AC1A/1(Efd) -> Efd/1
  Vstab/1 -> AC1A/4(Vstab)
  Ifd/1 -> AC1A/3(Ifd)
  Vt/1 -> AC1A/2(Vt)
  Vref/1 -> AC1A/1(Vref)
  Q_meas/1 -> AC1A/5(Q_meas)

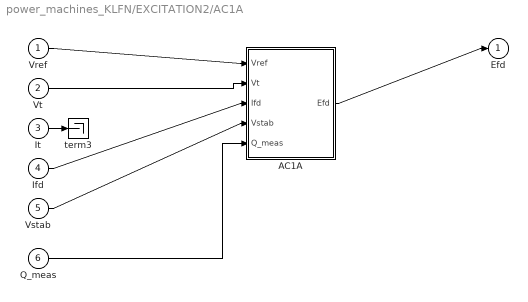
== system power_machines_KLFN/EXCITATION2/AC1A ==
  Vref : Inport
  Vt : Inport  Port=2
  It : Inport  Port=3
  Ifd : Inport  Port=4
  Vstab : Inport  Port=5
  Q_meas : Inport  Port=6
  AC1A : Subsystem  AncestorBlock=sps_avr/AC1A Excitation System  mask(AC1A Excitation System){Tr=20e-11, KaTa=[150 0.012], VAminmax=[-14.5 14.5], VRminmax=[-5.43 6.03], KfTf=[0.03 1.0], TbTc=[0 0], KeTe=[1.0 0.42], Ve12=[4.18 3.14], SeVe12=[0.10 0.03], Kd=0.38, Kc=0.20, v0=[1.0055 2.0057], TsBlock=-2}
      mask prompts: Tr "Low-pass filter time constant Tr(s):"; KaTa "Voltage regulator gain and time constant [Ka Ta(s)]:"; VAminmax "Voltage regulator internal limits [VAmin(pu) VAmax(pu)]:"; VRminmax "Voltage regulator output limits [VRmin(pu) VRmax(pu)]:"; KfTf "Damping filter gain and time constant [Kf Tf(s)]:"; TbTc "Transient gain reduction lead and lag time constants [Tb(s) Tc(s)]:"; KeTe "Exciter gain and time constant [Ke Te(s)]:"; Ve12 "Exciter alternator voltage values [Ve1(pu) Ve2(pu)]:"; SeVe12 "Exciter saturation function values [SeVe1(pu) SeVe2(pu)]:"; Kd "Demagnetizing factor Kd(pu):"; Kc "Rectifier loading factor Kc(pu):"; v0 "Initial values of terminal voltage and field voltage [Vt0(pu) Efd0(pu)]:"; TsBlock "Sample time:"
      mask help: Implements a synchronous machine voltage regulator and exciter based on the IEEE type AC1A excitation system model. The output is the field voltage to apply to the Vf input of a Synchronous Machine block. Inputs and output are in p.u.
      mask init: same as power_machines_KLFN/EXCITATION1/AC1A/AC1A
      mask Help: helpview(psbhelp);
      mask Display: color('blue');disp('AC1A')
  term3 : Terminator
  Efd : Outport
  wires:
  It/1 -> term3/1
  AC1A/1(Efd) -> Efd/1
  Vstab/1 -> AC1A/4(Vstab)
  Ifd/1 -> AC1A/3(Ifd)
  Vt/1 -> AC1A/2(Vt)
  Vref/1 -> AC1A/1(Vref)
  Q_meas/1 -> AC1A/5(Q_meas)

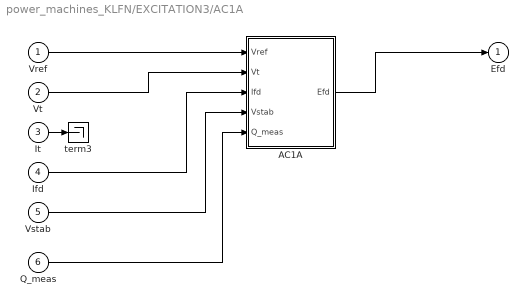
== system power_machines_KLFN/EXCITATION3/AC1A ==
  Vref : Inport
  Vt : Inport  Port=2
  It : Inport  Port=3
  Ifd : Inport  Port=4
  Vstab : Inport  Port=5
  Q_meas : Inport  Port=6
  AC1A : Subsystem  AncestorBlock=sps_avr/AC1A Excitation System  mask(AC1A Excitation System){Tr=20e-11, KaTa=[300 0.012], VAminmax=[-14.5 14.5], VRminmax=[-5.43 6.03], KfTf=[0.03 1.0], TbTc=[0 0], KeTe=[1.0 0.5], Ve12=[4.18 3.14], SeVe12=[0.10 0.03], Kd=0.38, Kc=0.20, v0=[1 2.1441], TsBlock=-2}
      mask prompts: Tr "Low-pass filter time constant Tr(s):"; KaTa "Voltage regulator gain and time constant [Ka Ta(s)]:"; VAminmax "Voltage regulator internal limits [VAmin(pu) VAmax(pu)]:"; VRminmax "Voltage regulator output limits [VRmin(pu) VRmax(pu)]:"; KfTf "Damping filter gain and time constant [Kf Tf(s)]:"; TbTc "Transient gain reduction lead and lag time constants [Tb(s) Tc(s)]:"; KeTe "Exciter gain and time constant [Ke Te(s)]:"; Ve12 "Exciter alternator voltage values [Ve1(pu) Ve2(pu)]:"; SeVe12 "Exciter saturation function values [SeVe1(pu) SeVe2(pu)]:"; Kd "Demagnetizing factor Kd(pu):"; Kc "Rectifier loading factor Kc(pu):"; v0 "Initial values of terminal voltage and field voltage [Vt0(pu) Efd0(pu)]:"; TsBlock "Sample time:"
      mask help: Implements a synchronous machine voltage regulator and exciter based on the IEEE type AC1A excitation system model. The output is the field voltage to apply to the Vf input of a Synchronous Machine block. Inputs and output are in p.u.
      mask init: same as power_machines_KLFN/EXCITATION1/AC1A/AC1A
      mask Help: helpview(psbhelp);
      mask Display: color('blue');disp('AC1A')
  term3 : Terminator
  Efd : Outport
  wires:
  It/1 -> term3/1
  AC1A/1(Efd) -> Efd/1
  Vstab/1 -> AC1A/4(Vstab)
  Ifd/1 -> AC1A/3(Ifd)
  Vt/1 -> AC1A/2(Vt)
  Vref/1 -> AC1A/1(Vref)
  Q_meas/1 -> AC1A/5(Q_meas)

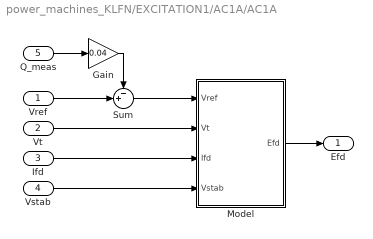
== system power_machines_KLFN/EXCITATION1/AC1A/AC1A ==
  Vref : Inport
  Vt : Inport  Port=2
  Ifd : Inport  Port=3
  Vstab : Inport  Port=4
  Q_meas : Inport  Port=5
  Gain : Gain  Gain=0.04
  Model : Subsystem  BlockChoice=Continuous
      link override Continuous/Vfe0//Ka: Value=Vfe0/Ka
      settings: AttributesFormatString=%<BlockChoice>  TemplateBlock=spsAC1AModel/Model  MemberBlocks=Continuous,Discrete
  Sum : Sum  Inputs=-+|
  Efd : Outport
  wires:
  Model/1(Efd) -> Efd/1
  Vstab/1 -> Model/4(Vstab)
  Ifd/1 -> Model/3(Ifd)
  Vt/1 -> Model/2(Vt)
  Vref/1 -> Sum/2
  Sum/1 -> Model/1(Vref)
  Q_meas/1 -> Gain/1
  Gain/1 -> Sum/1

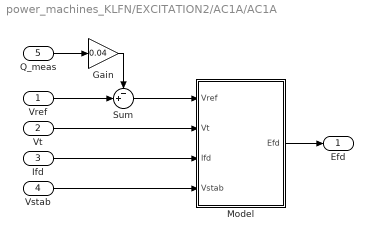
== system power_machines_KLFN/EXCITATION2/AC1A/AC1A ==
  Vref : Inport
  Vt : Inport  Port=2
  Ifd : Inport  Port=3
  Vstab : Inport  Port=4
  Q_meas : Inport  Port=5
  Gain : Gain  Gain=0.04
  Model : Subsystem  BlockChoice=Continuous
      link override Continuous/Vfe0//Ka: Value=Vfe0/Ka
      settings: AttributesFormatString=%<BlockChoice>  TemplateBlock=spsAC1AModel/Model  MemberBlocks=Continuous,Discrete
  Sum : Sum  Inputs=-+|
  Efd : Outport
  wires:
  Model/1(Efd) -> Efd/1
  Vstab/1 -> Model/4(Vstab)
  Ifd/1 -> Model/3(Ifd)
  Vt/1 -> Model/2(Vt)
  Vref/1 -> Sum/2
  Sum/1 -> Model/1(Vref)
  Q_meas/1 -> Gain/1
  Gain/1 -> Sum/1

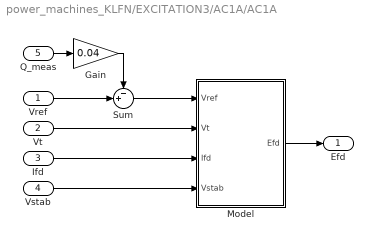
== system power_machines_KLFN/EXCITATION3/AC1A/AC1A ==
  Vref : Inport
  Vt : Inport  Port=2
  Ifd : Inport  Port=3
  Vstab : Inport  Port=4
  Q_meas : Inport  Port=5
  Gain : Gain  Gain=0.04
  Model : Subsystem  BlockChoice=Continuous
      link override Continuous/Vfe0//Ka: Value=Vfe0/Ka
      settings: AttributesFormatString=%<BlockChoice>  TemplateBlock=spsAC1AModel/Model  MemberBlocks=Continuous,Discrete
  Sum : Sum  Inputs=-+|
  Efd : Outport
  wires:
  Model/1(Efd) -> Efd/1
  Vstab/1 -> Model/4(Vstab)
  Ifd/1 -> Model/3(Ifd)
  Vt/1 -> Model/2(Vt)
  Vref/1 -> Sum/2
  Sum/1 -> Model/1(Vref)
  Q_meas/1 -> Gain/1
  Gain/1 -> Sum/1

== system power_machines_KLFN/EXCITATION1/AC1A/AC1A/Model ==
  Vref : Inport
  Vt : Inport  Port=2
  Ifd : Inport  Port=3
  Vstab : Inport  Port=4
  Continuous : spsAC1AModel/Continuous  SystemSampleTime=-1
  Efd : Outport
  wires:
  Vref/1 -> Continuous/1
  Vt/1 -> Continuous/2
  Ifd/1 -> Continuous/3
  Vstab/1 -> Continuous/4
  Continuous/1 -> Efd/1

== system power_machines_KLFN/EXCITATION2/AC1A/AC1A/Model ==
  Vref : Inport
  Vt : Inport  Port=2
  Ifd : Inport  Port=3
  Vstab : Inport  Port=4
  Continuous : spsAC1AModel/Continuous  SystemSampleTime=-1
  Efd : Outport
  wires:
  Vref/1 -> Continuous/1
  Vt/1 -> Continuous/2
  Ifd/1 -> Continuous/3
  Vstab/1 -> Continuous/4
  Continuous/1 -> Efd/1

== system power_machines_KLFN/EXCITATION3/AC1A/AC1A/Model ==
  Vref : Inport
  Vt : Inport  Port=2
  Ifd : Inport  Port=3
  Vstab : Inport  Port=4
  Continuous : spsAC1AModel/Continuous  SystemSampleTime=-1
  Efd : Outport
  wires:
  Vref/1 -> Continuous/1
  Vt/1 -> Continuous/2
  Ifd/1 -> Continuous/3
  Vstab/1 -> Continuous/4
  Continuous/1 -> Efd/1
